simulink model "Model"  (R2020b)
settings: Solver=VariableStepAuto  StartTime=0.0  StopTime=10.0  RelTol=1e-3
values from neighbouring files (symbols this model uses):
  theta1 = csi(1,1)    [F.m]
  theta2 = csi(2,1)    [F.m]
settings Model: Creator=daniele_ravasio  LastModifiedBy=daniele_ravasio

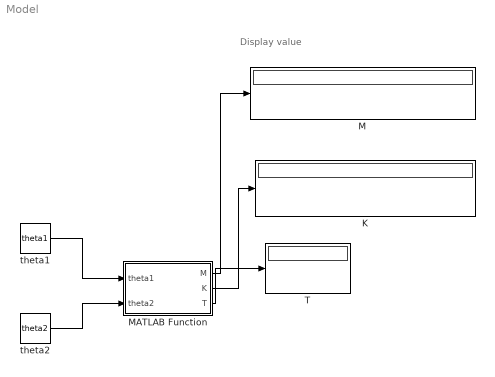
== system Model ==
  note: Display value
  K : Display
  M : Display
  MATLAB Function : MATLAB Function  TreatAsAtomicUnit=on
  T : Display
  theta1 : Constant  Value=theta1  VectorParams1D=off
  theta2 : Constant  Value=theta2  VectorParams1D=off
  wires:
  theta1/1 -> MATLAB Function/1(theta1)
  theta2/1 -> MATLAB Function/2(theta2)
  MATLAB Function/1(M) -> M/1
  MATLAB Function/3(T) -> T/1
  MATLAB Function/2(K) -> K/1

== matlab function Model/MATLAB Function ==
  data: theta1 input; M output; theta2 input; K output; T output
function [M,K,T] = fcn(theta1,theta2)

[PKM] = Define_Robot();

[M,K,T] = Matrici_Lagrange(PKM,theta1,theta2);

end
